simulink model "FO"  (R2014b)
settings: Solver=ode45  StartTime=0.0  StopTime=50  FixedStep=Ts  RelTol=1e-5
libraries: simulink x1
settings Model: Creator=dbr  LastModifiedBy=dbr
settings DataIOCC: SignalLoggingSaveFormat=ModelDataLogs
settings OptimizationCC: ExpressionDepthLimit=2147483647
settings DebuggingCC: AlgebraicLoopMsg=none  UnderspecifiedInitializationDetection=Classic  MergeDetectMultiDrivingBlocksExec=none  SolverPrmCheckMsg=none  FcnCallInpInsideContextMsg=EnableAllAsWarning  StateNameClashWarn=warning

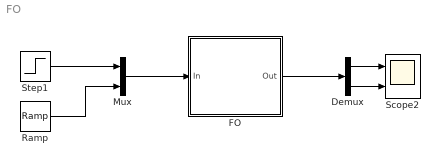
== system FO ==
  Demux : Demux  Outputs=2
  FO : Subsystem  mask(Discrete FO system: Euler Backward Difference (EBD) approximation method){Ts=0.05, K_P=1, T_lag=10}
      mask prompts: Ts "Sampling period Ts [s]"; K_P "Gain K_P"; T_lag "Time constant T_lag [s]"
  Mux : Mux  Inputs=2
  Ramp : simulink/Sources/Ramp  slope=0.1  start=2  X0=0
  Scope2 : Scope  NumInputPorts=2
      settings: TimeRange=50  YMin=-5~-5  YMax=5~5  SaveName=ScopeData2
  Step1 : Step
  wires:
  Step1/1 -> Mux/1
  Ramp/1 -> Mux/2
  Mux/1 -> FO/1(In)
  FO/1(Out) -> Demux/1
  Demux/2 -> Scope2/2
  Demux/1 -> Scope2/1

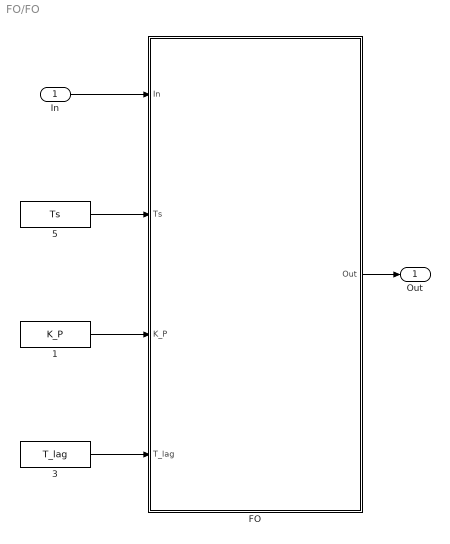
== system FO/FO ==
  In : Inport
  1 : Constant  Value=K_P
  3 : Constant  Value=T_lag
  5 : Constant  Value=Ts
  FO : MATLAB Function  TreatAsAtomicUnit=on  SystemSampleTime=Ts
  Out : Outport
  wires:
  FO/1(Out) -> Out/1
  In/1 -> FO/1(In)
  5/1 -> FO/2(Ts)
  1/1 -> FO/3(K_P)
  3/1 -> FO/4(T_lag)

== matlab function FO/FO ==
  data: In input; Ts input; K_P input; Out output; T_lag input
function Out = FO(In,Ts,K_P,T_lag)

persistent Out_p

if isempty(Out_p)
    Out_p = K_P*In;
end

% Euler backward
K = Ts/T_lag;
Out = (1/(1+K))*Out_p + K_P*(K/(1+K))*In;
Out_p = Out;
